simulink model "ThreeSines_DrSaher"  (R2018a)
settings: Solver=FixedStepDiscrete  StartTime=0.0  StopTime=0.1  RelTol=1e-3
InitFcn:
  | ST = 2e-8
  | Ts = 2e-8
libraries: simulink x10, hdlsllib x8, powerlib x1
(part 2 of 2)

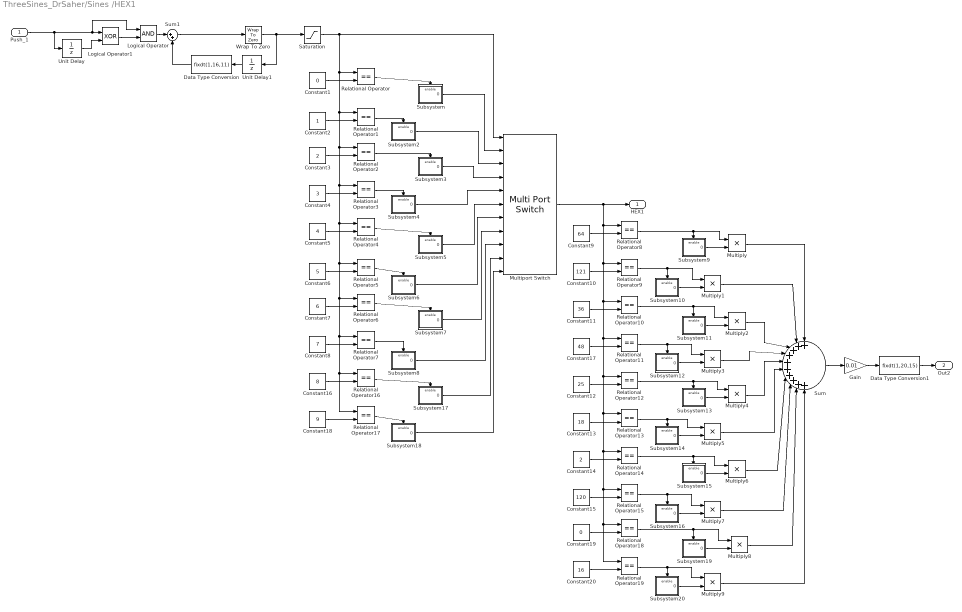
== system ThreeSines_DrSaher/Sines /HEX1 ==
  Push_1 : Inport
  Constant1 : Constant  Value=0  OutMax=[1]  OutDataTypeStr=fixdt(1,16,14)  SampleTime=Ts
  Constant10 : Constant  Value=121  OutMax=[121]  OutDataTypeStr=fixdt(0,7,0)  SampleTime=Ts
  Constant11 : Constant  Value=36  OutMax=[36]  OutDataTypeStr=fixdt(0,7,0)  SampleTime=Ts
  Constant12 : Constant  Value=25  OutMax=[25]  OutDataTypeStr=fixdt(0,7,0)  SampleTime=Ts
  Constant13 : Constant  Value=18  OutMax=[18]  OutDataTypeStr=fixdt(0,7,0)  SampleTime=Ts
  Constant14 : Constant  Value=2  OutMax=[2]  OutDataTypeStr=fixdt(0,7,0)  SampleTime=Ts
  Constant15 : Constant  Value=120  OutMax=[120]  OutDataTypeStr=fixdt(0,7,0)  SampleTime=Ts
  Constant16 : Constant  Value=8  OutMax=[8]  OutDataTypeStr=fixdt(1,16,11)  SampleTime=Ts
  Constant17 : Constant  Value=48  OutMax=[48]  OutDataTypeStr=fixdt(0,7,0)  SampleTime=Ts
  Constant18 : Constant  Value=9  OutMax=[9]  OutDataTypeStr=fixdt(1,16,11)  SampleTime=Ts
  Constant19 : Constant  Value=0  OutMax=[0]  OutDataTypeStr=fixdt(0,7,0)  SampleTime=Ts
  Constant2 : Constant  OutMax=[1]  OutDataTypeStr=fixdt(1,16,14)  SampleTime=Ts
  Constant20 : Constant  Value=16  OutMax=[16]  OutDataTypeStr=fixdt(0,7,0)  SampleTime=Ts
  Constant3 : Constant  Value=2  OutMax=[2]  OutDataTypeStr=fixdt(1,16,13)  SampleTime=Ts
  Constant4 : Constant  Value=3  OutMax=[3]  OutDataTypeStr=fixdt(1,16,13)  SampleTime=Ts
  Constant5 : Constant  Value=4  OutMax=[4]  OutDataTypeStr=fixdt(1,16,12)  SampleTime=Ts
  Constant6 : Constant  Value=5  OutMax=[5]  OutDataTypeStr=fixdt(1,16,12)  SampleTime=Ts
  Constant7 : Constant  Value=6  OutMax=[6]  OutDataTypeStr=fixdt(1,16,12)  SampleTime=Ts
  Constant8 : Constant  Value=7  OutMax=[7]  OutDataTypeStr=fixdt(1,16,12)  SampleTime=Ts
  Constant9 : Constant  Value=64  OutMax=[64]  OutDataTypeStr=fixdt(0,7,0)  SampleTime=Ts
  Data Type Conversion : DataTypeConversion  OutMax=[11]  OutDataTypeStr=fixdt(1,16,11)
  Data Type Conversion1 : DataTypeConversion  OutMin=[0]  OutMax=[0.09]  OutDataTypeStr=fixdt(1,20,15)
  Gain : Gain  Gain=0.01
  Logical Operator : Logic  AllPortsSameDT=off  OutDataTypeStr=boolean
  Logical Operator1 : Logic  Operator=XOR  AllPortsSameDT=off  OutDataTypeStr=boolean
  Multiply{,1..9} (10 alike) : Product
  Multiport Switch : MultiPortSwitch  DataPortOrder=Zero-based contiguous  Inputs=10  zeroidx=on
  Relational Operator{,1..19} (20 alike) : RelationalOperator  Operator===  OutDataTypeStr=boolean  RndMeth=Nearest
  Saturation : Saturate  UpperLimit=9  LowerLimit=0
  Subsystem : Subsystem
  Subsystem10 : Subsystem
  Subsystem11 : Subsystem
  Subsystem12 : Subsystem
  Subsystem13 : Subsystem
  Subsystem14 : Subsystem
  Subsystem15 : Subsystem
  Subsystem16 : Subsystem
  Subsystem17 : Subsystem
  Subsystem18 : Subsystem
  Subsystem19 : Subsystem
  Subsystem2 : Subsystem
  Subsystem20 : Subsystem
  Subsystem3 : Subsystem
  Subsystem4 : Subsystem
  Subsystem5 : Subsystem
  Subsystem6 : Subsystem
  Subsystem7 : Subsystem
  Subsystem8 : Subsystem
  Subsystem9 : Subsystem
  Sum : Sum  Inputs=10
  Sum1 : Sum  Inputs=|++
  Unit Delay : UnitDelay  SampleTime=Ts
  Unit Delay1 : UnitDelay  SampleTime=Ts
  Wrap To Zero : simulink/Discontinuities/Wrap To Zero  Threshold=9
      settings: SourceProductName=Simulink  SourceProductBaseCode=SL
  HEX1 : Outport
  Out2 : Outport  Port=2  OutMax=[0.9]
  wires:
  Sum/1 -> Gain/1
  Data Type Conversion/1 -> Sum1/2
  Wrap To Zero/1 -> Unit Delay1/1, Saturation/1
  Sum1/1 -> Wrap To Zero/1
  Unit Delay1/1 -> Data Type Conversion/1
  Logical Operator/1 -> Sum1/1
  Logical Operator1/1 -> Logical Operator/2
  Unit Delay/1 -> Logical Operator1/2
  Push_1/1 -> Logical Operator1/1, Logical Operator/1, Unit Delay/1
  Saturation/1 -> Multiport Switch/1, Relational Operator17/1, Relational Operator16/1, Relational Operator7/1, Relational Operator6/1, Relational Operator5/1, Relational Operator4/1, Relational Operator3/1, Relational Operator2/1, Relational Operator1/1, Relational Operator/1
  Subsystem17/1(0) -> Multiport Switch/10
  Relational Operator19/1 -> Multiply9/1, Subsystem20/Enable
  Subsystem13/1(0) -> Multiply4/2
  Relational Operator6/1 -> Subsystem7/Enable
  Constant9/1 -> Relational Operator8/2
  Subsystem6/1(0) -> Multiport Switch/7
  Constant14/1 -> Relational Operator14/2
  Relational Operator7/1 -> Subsystem8/Enable
  Relational Operator4/1 -> Subsystem5/Enable
  Relational Operator/1 -> Subsystem/Enable
  Subsystem2/1(0) -> Multiport Switch/3
  Relational Operator15/1 -> Multiply7/1, Subsystem16/Enable
  Multiply4/1 -> Sum/5
  Constant17/1 -> Relational Operator11/2
  Subsystem11/1(0) -> Multiply2/2
  Constant20/1 -> Relational Operator19/2
  Constant8/1 -> Relational Operator7/2
  Multiply9/1 -> Sum/10
  Constant10/1 -> Relational Operator9/2
  Constant13/1 -> Relational Operator13/2
  Subsystem5/1(0) -> Multiport Switch/6
  Subsystem8/1(0) -> Multiport Switch/9
  Relational Operator9/1 -> Subsystem10/Enable, Multiply1/1
  Relational Operator8/1 -> Subsystem9/Enable, Multiply/1
  Constant6/1 -> Relational Operator5/2
  Multiply7/1 -> Sum/8
  Constant15/1 -> Relational Operator15/2
  Multiply6/1 -> Sum/7
  Relational Operator14/1 -> Subsystem15/Enable, Multiply6/1
  Constant18/1 -> Relational Operator17/2
  Relational Operator12/1 -> Subsystem13/Enable, Multiply4/1
  Subsystem14/1(0) -> Multiply5/2
  Subsystem20/1(0) -> Multiply9/2
  Constant7/1 -> Relational Operator6/2
  Constant4/1 -> Relational Operator3/2
  Relational Operator1/1 -> Subsystem2/Enable
  Constant1/1 -> Relational Operator/2
  Relational Operator3/1 -> Subsystem4/Enable
  Relational Operator5/1 -> Subsystem6/Enable
  Subsystem3/1(0) -> Multiport Switch/4
  Constant2/1 -> Relational Operator1/2
  Constant5/1 -> Relational Operator4/2
  Relational Operator2/1 -> Subsystem3/Enable
  Constant12/1 -> Relational Operator12/2
  Multiply2/1 -> Sum/3
  Multiply8/1 -> Sum/9
  Subsystem4/1(0) -> Multiport Switch/5
  Relational Operator17/1 -> Subsystem18/Enable
  Constant3/1 -> Relational Operator2/2
  Subsystem7/1(0) -> Multiport Switch/8
  Constant19/1 -> Relational Operator18/2
  Multiply/1 -> Sum/1
  Multiport Switch/1 -> Relational Operator9/1, Relational Operator10/1, Relational Operator12/1, Relational Operator13/1, Relational Operator14/1, Relational Operator15/1, Relational Operator18/1, Relational Operator19/1, Relational Operator11/1, Relational Operator8/1, HEX1/1
  Multiply5/1 -> Sum/6
  Multiply1/1 -> Sum/2
  Relational Operator11/1 -> Subsystem12/Enable, Multiply3/1
  Constant11/1 -> Relational Operator10/2
  Subsystem12/1(0) -> Multiply3/2
  Subsystem9/1(0) -> Multiply/2
  Subsystem16/1(0) -> Multiply7/2
  Subsystem18/1(0) -> Multiport Switch/11
  Relational Operator13/1 -> Subsystem14/Enable, Multiply5/1
  Subsystem10/1(0) -> Multiply1/2
  Relational Operator18/1 -> Subsystem19/Enable, Multiply8/1
  Multiply3/1 -> Sum/4
  Subsystem19/1(0) -> Multiply8/2
  Subsystem15/1(0) -> Multiply6/2
  Relational Operator16/1 -> Subsystem17/Enable
  Subsystem/1(0) -> Multiport Switch/2
  Constant16/1 -> Relational Operator16/2
  Relational Operator10/1 -> Subsystem11/Enable, Multiply2/1
  Gain/1 -> Data Type Conversion1/1
  Data Type Conversion1/1 -> Out2/1

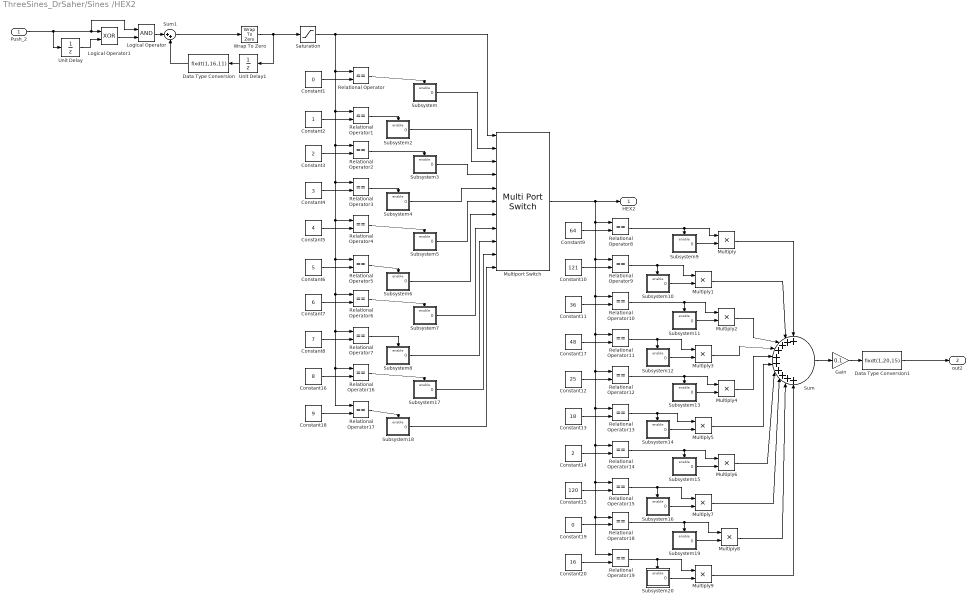
== system ThreeSines_DrSaher/Sines /HEX2 ==
  Push_2 : Inport
  Constant1 : Constant  Value=0  OutMax=[1]  OutDataTypeStr=fixdt(1,16,14)  SampleTime=Ts
  Constant10 : Constant  Value=121  OutMax=[121]  OutDataTypeStr=fixdt(0,7,0)  SampleTime=Ts
  Constant11 : Constant  Value=36  OutMax=[36]  OutDataTypeStr=fixdt(0,7,0)  SampleTime=Ts
  Constant12 : Constant  Value=25  OutMax=[25]  OutDataTypeStr=fixdt(0,7,0)  SampleTime=Ts
  Constant13 : Constant  Value=18  OutMax=[18]  OutDataTypeStr=fixdt(0,7,0)  SampleTime=Ts
  Constant14 : Constant  Value=2  OutMax=[2]  OutDataTypeStr=fixdt(0,7,0)  SampleTime=Ts
  Constant15 : Constant  Value=120  OutMax=[120]  OutDataTypeStr=fixdt(0,7,0)  SampleTime=Ts
  Constant16 : Constant  Value=8  OutMax=[8]  OutDataTypeStr=fixdt(1,16,11)  SampleTime=Ts
  Constant17 : Constant  Value=48  OutMax=[48]  OutDataTypeStr=fixdt(0,7,0)  SampleTime=Ts
  Constant18 : Constant  Value=9  OutMax=[9]  OutDataTypeStr=fixdt(1,16,11)  SampleTime=Ts
  Constant19 : Constant  Value=0  OutMax=[0]  OutDataTypeStr=fixdt(0,7,0)  SampleTime=Ts
  Constant2 : Constant  OutMax=[1]  OutDataTypeStr=fixdt(1,16,14)  SampleTime=Ts
  Constant20 : Constant  Value=16  OutMax=[16]  OutDataTypeStr=fixdt(0,7,0)  SampleTime=Ts
  Constant3 : Constant  Value=2  OutMax=[2]  OutDataTypeStr=fixdt(1,16,13)  SampleTime=Ts
  Constant4 : Constant  Value=3  OutMax=[3]  OutDataTypeStr=fixdt(1,16,13)  SampleTime=Ts
  Constant5 : Constant  Value=4  OutMax=[4]  OutDataTypeStr=fixdt(1,16,12)  SampleTime=Ts
  Constant6 : Constant  Value=5  OutMax=[5]  OutDataTypeStr=fixdt(1,16,12)  SampleTime=Ts
  Constant7 : Constant  Value=6  OutMax=[6]  OutDataTypeStr=fixdt(1,16,12)  SampleTime=Ts
  Constant8 : Constant  Value=7  OutMax=[7]  OutDataTypeStr=fixdt(1,16,12)  SampleTime=Ts
  Constant9 : Constant  Value=64  OutMax=[64]  OutDataTypeStr=fixdt(0,7,0)  SampleTime=Ts
  Data Type Conversion : DataTypeConversion  OutMax=[11]  OutDataTypeStr=fixdt(1,16,11)
  Data Type Conversion1 : DataTypeConversion  OutMin=[0]  OutMax=[0.9]  OutDataTypeStr=fixdt(1,20,15)
  Gain : Gain  Gain=0.1
  Logical Operator : Logic  AllPortsSameDT=off  OutDataTypeStr=boolean
  Logical Operator1 : Logic  Operator=XOR  AllPortsSameDT=off  OutDataTypeStr=boolean
  Multiply{,1..9} (10 alike) : Product
  Multiport Switch : MultiPortSwitch  DataPortOrder=Zero-based contiguous  Inputs=10  zeroidx=on
  Relational Operator{,1..19} (20 alike) : RelationalOperator  Operator===  OutDataTypeStr=boolean  RndMeth=Nearest
  Saturation : Saturate  UpperLimit=9  LowerLimit=0
  Subsystem : Subsystem
  Subsystem10 : Subsystem
  Subsystem11 : Subsystem
  Subsystem12 : Subsystem
  Subsystem13 : Subsystem
  Subsystem14 : Subsystem
  Subsystem15 : Subsystem
  Subsystem16 : Subsystem
  Subsystem17 : Subsystem
  Subsystem18 : Subsystem
  Subsystem19 : Subsystem
  Subsystem2 : Subsystem
  Subsystem20 : Subsystem
  Subsystem3 : Subsystem
  Subsystem4 : Subsystem
  Subsystem5 : Subsystem
  Subsystem6 : Subsystem
  Subsystem7 : Subsystem
  Subsystem8 : Subsystem
  Subsystem9 : Subsystem
  Sum : Sum  Inputs=10
  Sum1 : Sum  Inputs=|++
  Unit Delay : UnitDelay  SampleTime=Ts
  Unit Delay1 : UnitDelay  SampleTime=Ts
  Wrap To Zero : simulink/Discontinuities/Wrap To Zero  Threshold=9
      settings: SourceProductName=Simulink  SourceProductBaseCode=SL
  HEX2 : Outport
  out2 : Outport  Port=2  OutMax=[0.9]
  wires:
  Relational Operator10/1 -> Multiply2/1, Subsystem11/Enable
  Constant16/1 -> Relational Operator16/2
  Subsystem/1(0) -> Multiport Switch/2
  Relational Operator16/1 -> Subsystem17/Enable
  Subsystem15/1(0) -> Multiply6/2
  Subsystem19/1(0) -> Multiply8/2
  Multiply3/1 -> Sum/4
  Relational Operator18/1 -> Multiply8/1, Subsystem19/Enable
  Subsystem10/1(0) -> Multiply1/2
  Relational Operator13/1 -> Multiply5/1, Subsystem14/Enable
  Subsystem18/1(0) -> Multiport Switch/11
  Subsystem16/1(0) -> Multiply7/2
  Subsystem9/1(0) -> Multiply/2
  Subsystem12/1(0) -> Multiply3/2
  Constant11/1 -> Relational Operator10/2
  Relational Operator11/1 -> Multiply3/1, Subsystem12/Enable
  Multiply1/1 -> Sum/2
  Multiply5/1 -> Sum/6
  Multiport Switch/1 -> HEX2/1, Relational Operator8/1, Relational Operator11/1, Relational Operator19/1, Relational Operator18/1, Relational Operator15/1, Relational Operator14/1, Relational Operator13/1, Relational Operator12/1, Relational Operator10/1, Relational Operator9/1
  Multiply/1 -> Sum/1
  Constant19/1 -> Relational Operator18/2
  Subsystem7/1(0) -> Multiport Switch/8
  Constant3/1 -> Relational Operator2/2
  Relational Operator17/1 -> Subsystem18/Enable
  Subsystem4/1(0) -> Multiport Switch/5
  Multiply8/1 -> Sum/9
  Multiply2/1 -> Sum/3
  Constant12/1 -> Relational Operator12/2
  Relational Operator2/1 -> Subsystem3/Enable
  Constant5/1 -> Relational Operator4/2
  Constant2/1 -> Relational Operator1/2
  Subsystem3/1(0) -> Multiport Switch/4
  Relational Operator5/1 -> Subsystem6/Enable
  Relational Operator3/1 -> Subsystem4/Enable
  Constant1/1 -> Relational Operator/2
  Relational Operator1/1 -> Subsystem2/Enable
  Constant4/1 -> Relational Operator3/2
  Constant7/1 -> Relational Operator6/2
  Subsystem20/1(0) -> Multiply9/2
  Subsystem14/1(0) -> Multiply5/2
  Relational Operator12/1 -> Multiply4/1, Subsystem13/Enable
  Constant18/1 -> Relational Operator17/2
  Relational Operator14/1 -> Multiply6/1, Subsystem15/Enable
  Multiply6/1 -> Sum/7
  Constant15/1 -> Relational Operator15/2
  Multiply7/1 -> Sum/8
  Constant6/1 -> Relational Operator5/2
  Relational Operator8/1 -> Multiply/1, Subsystem9/Enable
  Relational Operator9/1 -> Multiply1/1, Subsystem10/Enable
  Subsystem8/1(0) -> Multiport Switch/9
  Subsystem5/1(0) -> Multiport Switch/6
  Constant13/1 -> Relational Operator13/2
  Constant10/1 -> Relational Operator9/2
  Multiply9/1 -> Sum/10
  Constant8/1 -> Relational Operator7/2
  Constant20/1 -> Relational Operator19/2
  Subsystem11/1(0) -> Multiply2/2
  Constant17/1 -> Relational Operator11/2
  Multiply4/1 -> Sum/5
  Relational Operator15/1 -> Subsystem16/Enable, Multiply7/1
  Subsystem2/1(0) -> Multiport Switch/3
  Relational Operator/1 -> Subsystem/Enable
  Relational Operator4/1 -> Subsystem5/Enable
  Relational Operator7/1 -> Subsystem8/Enable
  Constant14/1 -> Relational Operator14/2
  Subsystem6/1(0) -> Multiport Switch/7
  Constant9/1 -> Relational Operator8/2
  Relational Operator6/1 -> Subsystem7/Enable
  Subsystem13/1(0) -> Multiply4/2
  Relational Operator19/1 -> Subsystem20/Enable, Multiply9/1
  Subsystem17/1(0) -> Multiport Switch/10
  Saturation/1 -> Relational Operator/1, Relational Operator1/1, Relational Operator2/1, Relational Operator3/1, Relational Operator4/1, Relational Operator5/1, Relational Operator6/1, Relational Operator7/1, Relational Operator16/1, Relational Operator17/1, Multiport Switch/1
  Push_2/1 -> Unit Delay/1, Logical Operator/1, Logical Operator1/1
  Unit Delay/1 -> Logical Operator1/2
  Logical Operator1/1 -> Logical Operator/2
  Logical Operator/1 -> Sum1/1
  Unit Delay1/1 -> Data Type Conversion/1
  Sum1/1 -> Wrap To Zero/1
  Wrap To Zero/1 -> Saturation/1, Unit Delay1/1
  Data Type Conversion/1 -> Sum1/2
  Sum/1 -> Gain/1
  Gain/1 -> Data Type Conversion1/1
  Data Type Conversion1/1 -> out2/1

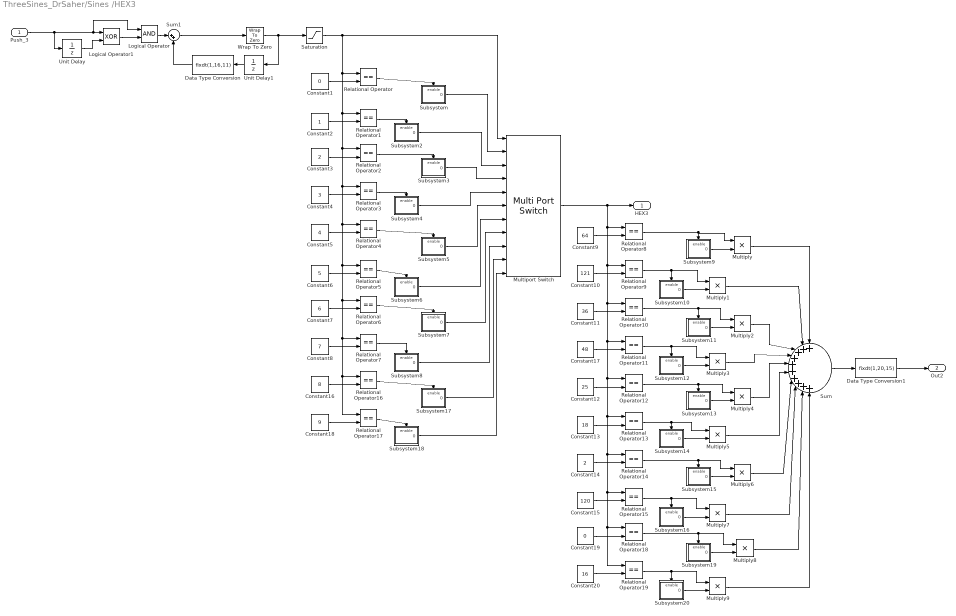
== system ThreeSines_DrSaher/Sines /HEX3 ==
  Push_3 : Inport
  Constant1 : Constant  Value=0  OutMax=[1]  OutDataTypeStr=fixdt(1,16,14)  SampleTime=Ts
  Constant10 : Constant  Value=121  OutMax=[121]  OutDataTypeStr=fixdt(0,7,0)  SampleTime=Ts
  Constant11 : Constant  Value=36  OutMax=[36]  OutDataTypeStr=fixdt(0,7,0)  SampleTime=Ts
  Constant12 : Constant  Value=25  OutMax=[25]  OutDataTypeStr=fixdt(0,7,0)  SampleTime=Ts
  Constant13 : Constant  Value=18  OutMax=[18]  OutDataTypeStr=fixdt(0,7,0)  SampleTime=Ts
  Constant14 : Constant  Value=2  OutMax=[2]  OutDataTypeStr=fixdt(0,7,0)  SampleTime=Ts
  Constant15 : Constant  Value=120  OutMax=[120]  OutDataTypeStr=fixdt(0,7,0)  SampleTime=Ts
  Constant16 : Constant  Value=8  OutMax=[8]  OutDataTypeStr=fixdt(1,16,11)  SampleTime=Ts
  Constant17 : Constant  Value=48  OutMax=[48]  OutDataTypeStr=fixdt(0,7,0)  SampleTime=Ts
  Constant18 : Constant  Value=9  OutMax=[9]  OutDataTypeStr=fixdt(1,16,11)  SampleTime=Ts
  Constant19 : Constant  Value=0  OutMax=[0]  OutDataTypeStr=fixdt(0,7,0)  SampleTime=Ts
  Constant2 : Constant  OutMax=[1]  OutDataTypeStr=fixdt(1,16,14)  SampleTime=Ts
  Constant20 : Constant  Value=16  OutMax=[16]  OutDataTypeStr=fixdt(0,7,0)  SampleTime=Ts
  Constant3 : Constant  Value=2  OutMax=[2]  OutDataTypeStr=fixdt(1,16,13)  SampleTime=Ts
  Constant4 : Constant  Value=3  OutMax=[3]  OutDataTypeStr=fixdt(1,16,13)  SampleTime=Ts
  Constant5 : Constant  Value=4  OutMax=[4]  OutDataTypeStr=fixdt(1,16,12)  SampleTime=Ts
  Constant6 : Constant  Value=5  OutMax=[5]  OutDataTypeStr=fixdt(1,16,12)  SampleTime=Ts
  Constant7 : Constant  Value=6  OutMax=[6]  OutDataTypeStr=fixdt(1,16,12)  SampleTime=Ts
  Constant8 : Constant  Value=7  OutMax=[7]  OutDataTypeStr=fixdt(1,16,12)  SampleTime=Ts
  Constant9 : Constant  Value=64  OutMax=[64]  OutDataTypeStr=fixdt(0,7,0)  SampleTime=Ts
  Data Type Conversion : DataTypeConversion  OutMax=[11]  OutDataTypeStr=fixdt(1,16,11)
  Data Type Conversion1 : DataTypeConversion  OutMin=[0]  OutMax=[9]  OutDataTypeStr=fixdt(1,20,15)
  Logical Operator : Logic  AllPortsSameDT=off  OutDataTypeStr=boolean
  Logical Operator1 : Logic  Operator=XOR  AllPortsSameDT=off  OutDataTypeStr=boolean
  Multiply{,1..9} (10 alike) : Product
  Multiport Switch : MultiPortSwitch  DataPortOrder=Zero-based contiguous  Inputs=10  zeroidx=on
  Relational Operator{,1..19} (20 alike) : RelationalOperator  Operator===  OutDataTypeStr=boolean  RndMeth=Nearest
  Saturation : Saturate  UpperLimit=9  LowerLimit=0
  Subsystem : Subsystem
  Subsystem10 : Subsystem
  Subsystem11 : Subsystem
  Subsystem12 : Subsystem
  Subsystem13 : Subsystem
  Subsystem14 : Subsystem
  Subsystem15 : Subsystem
  Subsystem16 : Subsystem
  Subsystem17 : Subsystem
  Subsystem18 : Subsystem
  Subsystem19 : Subsystem
  Subsystem2 : Subsystem
  Subsystem20 : Subsystem
  Subsystem3 : Subsystem
  Subsystem4 : Subsystem
  Subsystem5 : Subsystem
  Subsystem6 : Subsystem
  Subsystem7 : Subsystem
  Subsystem8 : Subsystem
  Subsystem9 : Subsystem
  Sum : Sum  Inputs=10
  Sum1 : Sum  Inputs=|++
  Unit Delay : UnitDelay  SampleTime=Ts
  Unit Delay1 : UnitDelay  SampleTime=Ts
  Wrap To Zero : simulink/Discontinuities/Wrap To Zero  Threshold=9
      settings: SourceProductName=Simulink  SourceProductBaseCode=SL
  HEX3 : Outport
  Out2 : Outport  Port=2  OutMax=[0.9]
  wires:
  Sum/1 -> Data Type Conversion1/1
  Data Type Conversion/1 -> Sum1/2
  Wrap To Zero/1 -> Unit Delay1/1, Saturation/1
  Sum1/1 -> Wrap To Zero/1
  Unit Delay1/1 -> Data Type Conversion/1
  Logical Operator/1 -> Sum1/1
  Logical Operator1/1 -> Logical Operator/2
  Unit Delay/1 -> Logical Operator1/2
  Push_3/1 -> Logical Operator1/1, Logical Operator/1, Unit Delay/1
  Saturation/1 -> Multiport Switch/1, Relational Operator17/1, Relational Operator16/1, Relational Operator7/1, Relational Operator6/1, Relational Operator5/1, Relational Operator4/1, Relational Operator3/1, Relational Operator2/1, Relational Operator1/1, Relational Operator/1
  Subsystem17/1(0) -> Multiport Switch/10
  Relational Operator19/1 -> Multiply9/1, Subsystem20/Enable
  Subsystem13/1(0) -> Multiply4/2
  Relational Operator6/1 -> Subsystem7/Enable
  Constant9/1 -> Relational Operator8/2
  Subsystem6/1(0) -> Multiport Switch/7
  Constant14/1 -> Relational Operator14/2
  Relational Operator7/1 -> Subsystem8/Enable
  Relational Operator4/1 -> Subsystem5/Enable
  Relational Operator/1 -> Subsystem/Enable
  Subsystem2/1(0) -> Multiport Switch/3
  Relational Operator15/1 -> Multiply7/1, Subsystem16/Enable
  Multiply4/1 -> Sum/5
  Constant17/1 -> Relational Operator11/2
  Subsystem11/1(0) -> Multiply2/2
  Constant20/1 -> Relational Operator19/2
  Constant8/1 -> Relational Operator7/2
  Multiply9/1 -> Sum/10
  Constant10/1 -> Relational Operator9/2
  Constant13/1 -> Relational Operator13/2
  Subsystem5/1(0) -> Multiport Switch/6
  Subsystem8/1(0) -> Multiport Switch/9
  Relational Operator9/1 -> Subsystem10/Enable, Multiply1/1
  Relational Operator8/1 -> Subsystem9/Enable, Multiply/1
  Constant6/1 -> Relational Operator5/2
  Multiply7/1 -> Sum/8
  Constant15/1 -> Relational Operator15/2
  Multiply6/1 -> Sum/7
  Relational Operator14/1 -> Subsystem15/Enable, Multiply6/1
  Constant18/1 -> Relational Operator17/2
  Relational Operator12/1 -> Subsystem13/Enable, Multiply4/1
  Subsystem14/1(0) -> Multiply5/2
  Subsystem20/1(0) -> Multiply9/2
  Constant7/1 -> Relational Operator6/2
  Constant4/1 -> Relational Operator3/2
  Relational Operator1/1 -> Subsystem2/Enable
  Constant1/1 -> Relational Operator/2
  Relational Operator3/1 -> Subsystem4/Enable
  Relational Operator5/1 -> Subsystem6/Enable
  Subsystem3/1(0) -> Multiport Switch/4
  Constant2/1 -> Relational Operator1/2
  Constant5/1 -> Relational Operator4/2
  Relational Operator2/1 -> Subsystem3/Enable
  Constant12/1 -> Relational Operator12/2
  Multiply2/1 -> Sum/3
  Multiply8/1 -> Sum/9
  Subsystem4/1(0) -> Multiport Switch/5
  Relational Operator17/1 -> Subsystem18/Enable
  Constant3/1 -> Relational Operator2/2
  Subsystem7/1(0) -> Multiport Switch/8
  Constant19/1 -> Relational Operator18/2
  Multiply/1 -> Sum/1
  Multiport Switch/1 -> Relational Operator9/1, Relational Operator10/1, Relational Operator12/1, Relational Operator13/1, Relational Operator14/1, Relational Operator15/1, Relational Operator18/1, Relational Operator19/1, Relational Operator11/1, Relational Operator8/1, HEX3/1
  Multiply5/1 -> Sum/6
  Multiply1/1 -> Sum/2
  Relational Operator11/1 -> Subsystem12/Enable, Multiply3/1
  Constant11/1 -> Relational Operator10/2
  Subsystem12/1(0) -> Multiply3/2
  Subsystem9/1(0) -> Multiply/2
  Subsystem16/1(0) -> Multiply7/2
  Subsystem18/1(0) -> Multiport Switch/11
  Relational Operator13/1 -> Subsystem14/Enable, Multiply5/1
  Subsystem10/1(0) -> Multiply1/2
  Relational Operator18/1 -> Subsystem19/Enable, Multiply8/1
  Multiply3/1 -> Sum/4
  Subsystem19/1(0) -> Multiply8/2
  Subsystem15/1(0) -> Multiply6/2
  Relational Operator16/1 -> Subsystem17/Enable
  Subsystem/1(0) -> Multiport Switch/2
  Constant16/1 -> Relational Operator16/2
  Relational Operator10/1 -> Subsystem11/Enable, Multiply2/1
  Data Type Conversion1/1 -> Out2/1

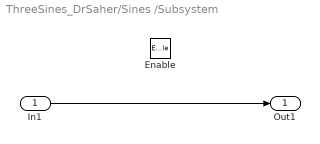
== system ThreeSines_DrSaher/Sines /Subsystem ==
  In1 : Inport
  Enable : EnablePort
  Out1 : Outport  InitialOutput=[0]
  wires:
  In1/1 -> Out1/1

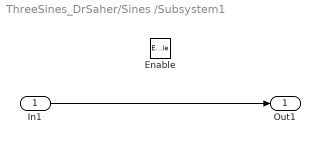
== system ThreeSines_DrSaher/Sines /Subsystem1 ==
  In1 : Inport
  Enable : EnablePort
  Out1 : Outport  InitialOutput=[0]
  wires:
  In1/1 -> Out1/1

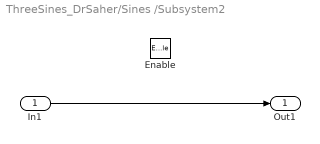
== system ThreeSines_DrSaher/Sines /Subsystem2 ==
  In1 : Inport
  Enable : EnablePort
  Out1 : Outport  InitialOutput=[0]
  wires:
  In1/1 -> Out1/1

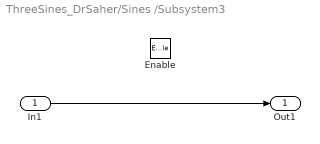
== system ThreeSines_DrSaher/Sines /Subsystem3 ==
  In1 : Inport
  Enable : EnablePort
  Out1 : Outport  InitialOutput=[0]
  wires:
  In1/1 -> Out1/1

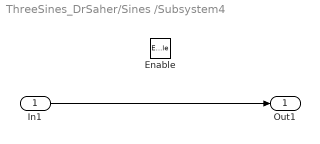
== system ThreeSines_DrSaher/Sines /Subsystem4 ==
  In1 : Inport
  Enable : EnablePort
  Out1 : Outport  InitialOutput=[0]
  wires:
  In1/1 -> Out1/1

== system ThreeSines_DrSaher/Sines /Subsystem5 ==
  In1 : Inport
  Enable : EnablePort
  Out1 : Outport  InitialOutput=[0]
  wires:
  In1/1 -> Out1/1

== system ThreeSines_DrSaher/Sines /Subsystem6 ==
  In1 : Inport
  Enable : EnablePort
  Out1 : Outport  InitialOutput=[0]
  wires:
  In1/1 -> Out1/1

== system ThreeSines_DrSaher/Sines /Subsystem7 ==
  In1 : Inport
  Enable : EnablePort
  Out1 : Outport  InitialOutput=[0]
  wires:
  In1/1 -> Out1/1

== system ThreeSines_DrSaher/Sines /aPA_Save ==
  MulNumber : Inport
  Enable : EnablePort
  MulResult : Outport  InitialOutput=[0]
  wires:
  MulNumber/1 -> MulResult/1

== system ThreeSines_DrSaher/Sines /aPA_Save1 ==
  MulNumber : Inport
  Enable : EnablePort
  MulResult : Outport  InitialOutput=[0]
  wires:
  MulNumber/1 -> MulResult/1

== system ThreeSines_DrSaher/Sines /aPA_Save2 ==
  MulNumber : Inport
  Enable : EnablePort
  MulResult : Outport  InitialOutput=[0]
  wires:
  MulNumber/1 -> MulResult/1

== system ThreeSines_DrSaher/Sines /bPA_Save ==
  MulNumber : Inport
  Enable : EnablePort
  MulResult : Outport  InitialOutput=[0]
  wires:
  MulNumber/1 -> MulResult/1

== system ThreeSines_DrSaher/Sines /bPA_Save1 ==
  MulNumber : Inport
  Enable : EnablePort
  MulResult : Outport  InitialOutput=[0]
  wires:
  MulNumber/1 -> MulResult/1

== system ThreeSines_DrSaher/Sines /bPA_Save2 ==
  MulNumber : Inport
  Enable : EnablePort
  MulResult : Outport  InitialOutput=[0]
  wires:
  MulNumber/1 -> MulResult/1

== system ThreeSines_DrSaher/Sines /cPA_Save ==
  MulNumber : Inport
  Enable : EnablePort
  MulResult : Outport  InitialOutput=[0]
  wires:
  MulNumber/1 -> MulResult/1

== system ThreeSines_DrSaher/Sines /cPA_Save1 ==
  MulNumber : Inport
  Enable : EnablePort
  MulResult : Outport  InitialOutput=[0]
  wires:
  MulNumber/1 -> MulResult/1

== system ThreeSines_DrSaher/Sines /cPA_Save2 ==
  MulNumber : Inport
  Enable : EnablePort
  MulResult : Outport  InitialOutput=[0]
  wires:
  MulNumber/1 -> MulResult/1

== system ThreeSines_DrSaher/Sines /dPA_Save ==
  MulNumber : Inport
  Enable : EnablePort
  MulResult : Outport  InitialOutput=[0]
  wires:
  MulNumber/1 -> MulResult/1

== system ThreeSines_DrSaher/Sines /dPA_Save1 ==
  MulNumber : Inport
  Enable : EnablePort
  MulResult : Outport  InitialOutput=[0]
  wires:
  MulNumber/1 -> MulResult/1

== system ThreeSines_DrSaher/Sines /dPA_Save2 ==
  MulNumber : Inport
  Enable : EnablePort
  MulResult : Outport  InitialOutput=[0]
  wires:
  MulNumber/1 -> MulResult/1

== system ThreeSines_DrSaher/Sines /HEX0/Subsystem ==
  Enable : EnablePort
  Constant9 : Constant  Value=64  OutMax=[64]  OutDataTypeStr=fixdt(0,7,0)  SampleTime=Ts
  0 : Outport  InitialOutput=[0]
  wires:
  Constant9/1 -> 0/1

== system ThreeSines_DrSaher/Sines /HEX0/Subsystem10 ==
  Enable : EnablePort
  Constant9 : Constant  OutMax=[1]  OutDataTypeStr=fixdt(1,16,14)  SampleTime=Ts
  0 : Outport  InitialOutput=[0]
  wires:
  Constant9/1 -> 0/1

== system ThreeSines_DrSaher/Sines /HEX0/Subsystem11 ==
  Enable : EnablePort
  Constant9 : Constant  Value=2  OutMax=[2]  OutDataTypeStr=fixdt(1,16,13)  SampleTime=Ts
  0 : Outport  InitialOutput=[0]
  wires:
  Constant9/1 -> 0/1

== system ThreeSines_DrSaher/Sines /HEX0/Subsystem12 ==
  Enable : EnablePort
  Constant9 : Constant  Value=3  VectorParams1D=off  OutMax=[3]  OutDataTypeStr=fixdt(1,16,13)  SampleTime=Ts
  0 : Outport  InitialOutput=[0]
  wires:
  Constant9/1 -> 0/1

== system ThreeSines_DrSaher/Sines /HEX0/Subsystem13 ==
  Enable : EnablePort
  Constant9 : Constant  Value=4  OutMax=[4]  OutDataTypeStr=fixdt(1,16,12)  SampleTime=Ts
  0 : Outport  InitialOutput=[0]
  wires:
  Constant9/1 -> 0/1

== system ThreeSines_DrSaher/Sines /HEX0/Subsystem14 ==
  Enable : EnablePort
  Constant9 : Constant  Value=5  OutMax=[5]  OutDataTypeStr=fixdt(1,16,12)  SampleTime=Ts
  0 : Outport  InitialOutput=[0]
  wires:
  Constant9/1 -> 0/1

== system ThreeSines_DrSaher/Sines /HEX0/Subsystem15 ==
  Enable : EnablePort
  Constant9 : Constant  Value=6  OutMax=[6]  OutDataTypeStr=fixdt(1,16,12)  SampleTime=Ts
  0 : Outport  InitialOutput=[0]
  wires:
  Constant9/1 -> 0/1

== system ThreeSines_DrSaher/Sines /HEX0/Subsystem16 ==
  Enable : EnablePort
  Constant9 : Constant  Value=7  OutMax=[7]  OutDataTypeStr=fixdt(1,16,12)  SampleTime=Ts
  0 : Outport  InitialOutput=[0]
  wires:
  Constant9/1 -> 0/1

== system ThreeSines_DrSaher/Sines /HEX0/Subsystem17 ==
  Enable : EnablePort
  Constant9 : Constant  Value=0  OutMax=[0]  OutDataTypeStr=fixdt(0,7,0)  SampleTime=Ts
  0 : Outport  InitialOutput=[0]
  wires:
  Constant9/1 -> 0/1

== system ThreeSines_DrSaher/Sines /HEX0/Subsystem18 ==
  Enable : EnablePort
  Constant9 : Constant  Value=16  OutMax=[16]  OutDataTypeStr=fixdt(0,7,0)  SampleTime=Ts
  0 : Outport  InitialOutput=[0]
  wires:
  Constant9/1 -> 0/1

== system ThreeSines_DrSaher/Sines /HEX0/Subsystem19 ==
  Enable : EnablePort
  Constant9 : Constant  Value=8  OutMax=[8]  OutDataTypeStr=fixdt(1,16,11)  SampleTime=Ts
  0 : Outport  InitialOutput=[0]
  wires:
  Constant9/1 -> 0/1

== system ThreeSines_DrSaher/Sines /HEX0/Subsystem2 ==
  Enable : EnablePort
  Constant9 : Constant  Value=121  OutMax=[121]  OutDataTypeStr=fixdt(0,7,0)  SampleTime=Ts
  0 : Outport  InitialOutput=[0]
  wires:
  Constant9/1 -> 0/1

== system ThreeSines_DrSaher/Sines /HEX0/Subsystem20 ==
  Enable : EnablePort
  Constant9 : Constant  Value=9  OutMax=[9]  OutDataTypeStr=fixdt(1,16,11)  SampleTime=Ts
  0 : Outport  InitialOutput=[0]
  wires:
  Constant9/1 -> 0/1

== system ThreeSines_DrSaher/Sines /HEX0/Subsystem3 ==
  Enable : EnablePort
  Constant9 : Constant  Value=36  OutMax=[36]  OutDataTypeStr=fixdt(0,7,0)  SampleTime=Ts
  0 : Outport  InitialOutput=[0]
  wires:
  Constant9/1 -> 0/1

== system ThreeSines_DrSaher/Sines /HEX0/Subsystem4 ==
  Enable : EnablePort
  Constant9 : Constant  Value=48  OutMax=[48]  OutDataTypeStr=fixdt(0,7,0)  SampleTime=Ts
  0 : Outport  InitialOutput=[0]
  wires:
  Constant9/1 -> 0/1

== system ThreeSines_DrSaher/Sines /HEX0/Subsystem5 ==
  Enable : EnablePort
  Constant9 : Constant  Value=25  OutMax=[25]  OutDataTypeStr=fixdt(0,7,0)  SampleTime=Ts
  0 : Outport  InitialOutput=[0]
  wires:
  Constant9/1 -> 0/1

== system ThreeSines_DrSaher/Sines /HEX0/Subsystem6 ==
  Enable : EnablePort
  Constant9 : Constant  Value=18  OutMax=[18]  OutDataTypeStr=fixdt(0,7,0)  SampleTime=Ts
  0 : Outport  InitialOutput=[0]
  wires:
  Constant9/1 -> 0/1

== system ThreeSines_DrSaher/Sines /HEX0/Subsystem7 ==
  Enable : EnablePort
  Constant9 : Constant  Value=2  OutMax=[2]  OutDataTypeStr=fixdt(0,7,0)  SampleTime=Ts
  0 : Outport  InitialOutput=[0]
  wires:
  Constant9/1 -> 0/1

== system ThreeSines_DrSaher/Sines /HEX0/Subsystem8 ==
  Enable : EnablePort
  Constant9 : Constant  Value=120  OutMax=[120]  OutDataTypeStr=fixdt(0,7,0)  SampleTime=Ts
  0 : Outport  InitialOutput=[0]
  wires:
  Constant9/1 -> 0/1

== system ThreeSines_DrSaher/Sines /HEX0/Subsystem9 ==
  Enable : EnablePort
  Constant9 : Constant  Value=0  OutMax=[0]  OutDataTypeStr=fixdt(1,16,10)  SampleTime=Ts
  0 : Outport  InitialOutput=[0]
  wires:
  Constant9/1 -> 0/1

== system ThreeSines_DrSaher/Sines /HEX1/Subsystem ==
  Enable : EnablePort
  Constant9 : Constant  Value=64  OutMax=[64]  OutDataTypeStr=fixdt(0,7,0)  SampleTime=Ts
  0 : Outport  InitialOutput=[0]
  wires:
  Constant9/1 -> 0/1

== system ThreeSines_DrSaher/Sines /HEX1/Subsystem10 ==
  Enable : EnablePort
  Constant9 : Constant  OutMax=[1]  OutDataTypeStr=fixdt(1,16,14)  SampleTime=Ts
  0 : Outport  InitialOutput=[0]
  wires:
  Constant9/1 -> 0/1

== system ThreeSines_DrSaher/Sines /HEX1/Subsystem11 ==
  Enable : EnablePort
  Constant9 : Constant  Value=2  OutMax=[2]  OutDataTypeStr=fixdt(1,16,13)  SampleTime=Ts
  0 : Outport  InitialOutput=[0]
  wires:
  Constant9/1 -> 0/1

== system ThreeSines_DrSaher/Sines /HEX1/Subsystem12 ==
  Enable : EnablePort
  Constant9 : Constant  Value=3  VectorParams1D=off  OutMax=[3]  OutDataTypeStr=fixdt(1,16,13)  SampleTime=Ts
  0 : Outport  InitialOutput=[0]
  wires:
  Constant9/1 -> 0/1

== system ThreeSines_DrSaher/Sines /HEX1/Subsystem13 ==
  Enable : EnablePort
  Constant9 : Constant  Value=4  OutMax=[4]  OutDataTypeStr=fixdt(1,16,12)  SampleTime=Ts
  0 : Outport  InitialOutput=[0]
  wires:
  Constant9/1 -> 0/1

== system ThreeSines_DrSaher/Sines /HEX1/Subsystem14 ==
  Enable : EnablePort
  Constant9 : Constant  Value=5  OutMax=[5]  OutDataTypeStr=fixdt(1,16,12)  SampleTime=Ts
  0 : Outport  InitialOutput=[0]
  wires:
  Constant9/1 -> 0/1

== system ThreeSines_DrSaher/Sines /HEX1/Subsystem15 ==
  Enable : EnablePort
  Constant9 : Constant  Value=6  OutMax=[6]  OutDataTypeStr=fixdt(1,16,12)  SampleTime=Ts
  0 : Outport  InitialOutput=[0]
  wires:
  Constant9/1 -> 0/1

== system ThreeSines_DrSaher/Sines /HEX1/Subsystem16 ==
  Enable : EnablePort
  Constant9 : Constant  Value=7  OutMax=[7]  OutDataTypeStr=fixdt(1,16,12)  SampleTime=Ts
  0 : Outport  InitialOutput=[0]
  wires:
  Constant9/1 -> 0/1

== system ThreeSines_DrSaher/Sines /HEX1/Subsystem17 ==
  Enable : EnablePort
  Constant9 : Constant  Value=0  OutMax=[0]  OutDataTypeStr=fixdt(0,7,0)  SampleTime=Ts
  0 : Outport  InitialOutput=[0]
  wires:
  Constant9/1 -> 0/1

== system ThreeSines_DrSaher/Sines /HEX1/Subsystem18 ==
  Enable : EnablePort
  Constant9 : Constant  Value=16  OutMax=[16]  OutDataTypeStr=fixdt(0,7,0)  SampleTime=Ts
  0 : Outport  InitialOutput=[0]
  wires:
  Constant9/1 -> 0/1

== system ThreeSines_DrSaher/Sines /HEX1/Subsystem19 ==
  Enable : EnablePort
  Constant9 : Constant  Value=8  OutMax=[8]  OutDataTypeStr=fixdt(1,16,11)  SampleTime=Ts
  0 : Outport  InitialOutput=[0]
  wires:
  Constant9/1 -> 0/1

== system ThreeSines_DrSaher/Sines /HEX1/Subsystem2 ==
  Enable : EnablePort
  Constant9 : Constant  Value=121  OutMax=[121]  OutDataTypeStr=fixdt(0,7,0)  SampleTime=Ts
  0 : Outport  InitialOutput=[0]
  wires:
  Constant9/1 -> 0/1

== system ThreeSines_DrSaher/Sines /HEX1/Subsystem20 ==
  Enable : EnablePort
  Constant9 : Constant  Value=9  OutMax=[9]  OutDataTypeStr=fixdt(1,16,11)  SampleTime=Ts
  0 : Outport  InitialOutput=[0]
  wires:
  Constant9/1 -> 0/1

== system ThreeSines_DrSaher/Sines /HEX1/Subsystem3 ==
  Enable : EnablePort
  Constant9 : Constant  Value=36  OutMax=[36]  OutDataTypeStr=fixdt(0,7,0)  SampleTime=Ts
  0 : Outport  InitialOutput=[0]
  wires:
  Constant9/1 -> 0/1

== system ThreeSines_DrSaher/Sines /HEX1/Subsystem4 ==
  Enable : EnablePort
  Constant9 : Constant  Value=48  OutMax=[48]  OutDataTypeStr=fixdt(0,7,0)  SampleTime=Ts
  0 : Outport  InitialOutput=[0]
  wires:
  Constant9/1 -> 0/1

== system ThreeSines_DrSaher/Sines /HEX1/Subsystem5 ==
  Enable : EnablePort
  Constant9 : Constant  Value=25  OutMax=[25]  OutDataTypeStr=fixdt(0,7,0)  SampleTime=Ts
  0 : Outport  InitialOutput=[0]
  wires:
  Constant9/1 -> 0/1

== system ThreeSines_DrSaher/Sines /HEX1/Subsystem6 ==
  Enable : EnablePort
  Constant9 : Constant  Value=18  OutMax=[18]  OutDataTypeStr=fixdt(0,7,0)  SampleTime=Ts
  0 : Outport  InitialOutput=[0]
  wires:
  Constant9/1 -> 0/1

== system ThreeSines_DrSaher/Sines /HEX1/Subsystem7 ==
  Enable : EnablePort
  Constant9 : Constant  Value=2  OutMax=[2]  OutDataTypeStr=fixdt(0,7,0)  SampleTime=Ts
  0 : Outport  InitialOutput=[0]
  wires:
  Constant9/1 -> 0/1

== system ThreeSines_DrSaher/Sines /HEX1/Subsystem8 ==
  Enable : EnablePort
  Constant9 : Constant  Value=120  OutMax=[120]  OutDataTypeStr=fixdt(0,7,0)  SampleTime=Ts
  0 : Outport  InitialOutput=[0]
  wires:
  Constant9/1 -> 0/1

== system ThreeSines_DrSaher/Sines /HEX1/Subsystem9 ==
  Enable : EnablePort
  Constant9 : Constant  Value=0  OutMax=[0]  OutDataTypeStr=fixdt(1,16,10)  SampleTime=Ts
  0 : Outport  InitialOutput=[0]
  wires:
  Constant9/1 -> 0/1

== system ThreeSines_DrSaher/Sines /HEX2/Subsystem ==
  Enable : EnablePort
  Constant9 : Constant  Value=64  OutMax=[64]  OutDataTypeStr=fixdt(0,7,0)  SampleTime=Ts
  0 : Outport  InitialOutput=[0]
  wires:
  Constant9/1 -> 0/1

== system ThreeSines_DrSaher/Sines /HEX2/Subsystem10 ==
  Enable : EnablePort
  Constant9 : Constant  OutMax=[1]  OutDataTypeStr=fixdt(1,16,14)  SampleTime=Ts
  0 : Outport  InitialOutput=[0]
  wires:
  Constant9/1 -> 0/1

== system ThreeSines_DrSaher/Sines /HEX2/Subsystem11 ==
  Enable : EnablePort
  Constant9 : Constant  Value=2  OutMax=[2]  OutDataTypeStr=fixdt(1,16,13)  SampleTime=Ts
  0 : Outport  InitialOutput=[0]
  wires:
  Constant9/1 -> 0/1

== system ThreeSines_DrSaher/Sines /HEX2/Subsystem12 ==
  Enable : EnablePort
  Constant9 : Constant  Value=3  VectorParams1D=off  OutMax=[3]  OutDataTypeStr=fixdt(1,16,13)  SampleTime=Ts
  0 : Outport  InitialOutput=[0]
  wires:
  Constant9/1 -> 0/1

== system ThreeSines_DrSaher/Sines /HEX2/Subsystem13 ==
  Enable : EnablePort
  Constant9 : Constant  Value=4  OutMax=[4]  OutDataTypeStr=fixdt(1,16,12)  SampleTime=Ts
  0 : Outport  InitialOutput=[0]
  wires:
  Constant9/1 -> 0/1

== system ThreeSines_DrSaher/Sines /HEX2/Subsystem14 ==
  Enable : EnablePort
  Constant9 : Constant  Value=5  OutMax=[5]  OutDataTypeStr=fixdt(1,16,12)  SampleTime=Ts
  0 : Outport  InitialOutput=[0]
  wires:
  Constant9/1 -> 0/1

== system ThreeSines_DrSaher/Sines /HEX2/Subsystem15 ==
  Enable : EnablePort
  Constant9 : Constant  Value=6  OutMax=[6]  OutDataTypeStr=fixdt(1,16,12)  SampleTime=Ts
  0 : Outport  InitialOutput=[0]
  wires:
  Constant9/1 -> 0/1

== system ThreeSines_DrSaher/Sines /HEX2/Subsystem16 ==
  Enable : EnablePort
  Constant9 : Constant  Value=7  OutMax=[7]  OutDataTypeStr=fixdt(1,16,12)  SampleTime=Ts
  0 : Outport  InitialOutput=[0]
  wires:
  Constant9/1 -> 0/1

== system ThreeSines_DrSaher/Sines /HEX2/Subsystem17 ==
  Enable : EnablePort
  Constant9 : Constant  Value=0  OutMax=[0]  OutDataTypeStr=fixdt(0,7,0)  SampleTime=Ts
  0 : Outport  InitialOutput=[0]
  wires:
  Constant9/1 -> 0/1

== system ThreeSines_DrSaher/Sines /HEX2/Subsystem18 ==
  Enable : EnablePort
  Constant9 : Constant  Value=16  OutMax=[16]  OutDataTypeStr=fixdt(0,7,0)  SampleTime=Ts
  0 : Outport  InitialOutput=[0]
  wires:
  Constant9/1 -> 0/1

== system ThreeSines_DrSaher/Sines /HEX2/Subsystem19 ==
  Enable : EnablePort
  Constant9 : Constant  Value=8  OutMax=[8]  OutDataTypeStr=fixdt(1,16,11)  SampleTime=Ts
  0 : Outport  InitialOutput=[0]
  wires:
  Constant9/1 -> 0/1

== system ThreeSines_DrSaher/Sines /HEX2/Subsystem2 ==
  Enable : EnablePort
  Constant9 : Constant  Value=121  OutMax=[121]  OutDataTypeStr=fixdt(0,7,0)  SampleTime=Ts
  0 : Outport  InitialOutput=[0]
  wires:
  Constant9/1 -> 0/1

== system ThreeSines_DrSaher/Sines /HEX2/Subsystem20 ==
  Enable : EnablePort
  Constant9 : Constant  Value=9  OutMax=[9]  OutDataTypeStr=fixdt(1,16,11)  SampleTime=Ts
  0 : Outport  InitialOutput=[0]
  wires:
  Constant9/1 -> 0/1

== system ThreeSines_DrSaher/Sines /HEX2/Subsystem3 ==
  Enable : EnablePort
  Constant9 : Constant  Value=36  OutMax=[36]  OutDataTypeStr=fixdt(0,7,0)  SampleTime=Ts
  0 : Outport  InitialOutput=[0]
  wires:
  Constant9/1 -> 0/1

== system ThreeSines_DrSaher/Sines /HEX2/Subsystem4 ==
  Enable : EnablePort
  Constant9 : Constant  Value=48  OutMax=[48]  OutDataTypeStr=fixdt(0,7,0)  SampleTime=Ts
  0 : Outport  InitialOutput=[0]
  wires:
  Constant9/1 -> 0/1

== system ThreeSines_DrSaher/Sines /HEX2/Subsystem5 ==
  Enable : EnablePort
  Constant9 : Constant  Value=25  OutMax=[25]  OutDataTypeStr=fixdt(0,7,0)  SampleTime=Ts
  0 : Outport  InitialOutput=[0]
  wires:
  Constant9/1 -> 0/1

== system ThreeSines_DrSaher/Sines /HEX2/Subsystem6 ==
  Enable : EnablePort
  Constant9 : Constant  Value=18  OutMax=[18]  OutDataTypeStr=fixdt(0,7,0)  SampleTime=Ts
  0 : Outport  InitialOutput=[0]
  wires:
  Constant9/1 -> 0/1

== system ThreeSines_DrSaher/Sines /HEX2/Subsystem7 ==
  Enable : EnablePort
  Constant9 : Constant  Value=2  OutMax=[2]  OutDataTypeStr=fixdt(0,7,0)  SampleTime=Ts
  0 : Outport  InitialOutput=[0]
  wires:
  Constant9/1 -> 0/1

== system ThreeSines_DrSaher/Sines /HEX2/Subsystem8 ==
  Enable : EnablePort
  Constant9 : Constant  Value=120  OutMax=[120]  OutDataTypeStr=fixdt(0,7,0)  SampleTime=Ts
  0 : Outport  InitialOutput=[0]
  wires:
  Constant9/1 -> 0/1

== system ThreeSines_DrSaher/Sines /HEX2/Subsystem9 ==
  Enable : EnablePort
  Constant9 : Constant  Value=0  OutMax=[0]  OutDataTypeStr=fixdt(1,16,10)  SampleTime=Ts
  0 : Outport  InitialOutput=[0]
  wires:
  Constant9/1 -> 0/1

== system ThreeSines_DrSaher/Sines /HEX3/Subsystem ==
  Enable : EnablePort
  Constant9 : Constant  Value=64  OutMax=[64]  OutDataTypeStr=fixdt(0,7,0)  SampleTime=Ts
  0 : Outport  InitialOutput=[0]
  wires:
  Constant9/1 -> 0/1

== system ThreeSines_DrSaher/Sines /HEX3/Subsystem10 ==
  Enable : EnablePort
  Constant9 : Constant  OutMax=[1]  OutDataTypeStr=fixdt(1,16,14)  SampleTime=Ts
  0 : Outport  InitialOutput=[0]
  wires:
  Constant9/1 -> 0/1

== system ThreeSines_DrSaher/Sines /HEX3/Subsystem11 ==
  Enable : EnablePort
  Constant9 : Constant  Value=2  OutMax=[2]  OutDataTypeStr=fixdt(1,16,13)  SampleTime=Ts
  0 : Outport  InitialOutput=[0]
  wires:
  Constant9/1 -> 0/1

== system ThreeSines_DrSaher/Sines /HEX3/Subsystem12 ==
  Enable : EnablePort
  Constant9 : Constant  Value=3  VectorParams1D=off  OutMax=[3]  OutDataTypeStr=fixdt(1,16,13)  SampleTime=Ts
  0 : Outport  InitialOutput=[0]
  wires:
  Constant9/1 -> 0/1

== system ThreeSines_DrSaher/Sines /HEX3/Subsystem13 ==
  Enable : EnablePort
  Constant9 : Constant  Value=4  OutMax=[4]  OutDataTypeStr=fixdt(1,16,12)  SampleTime=Ts
  0 : Outport  InitialOutput=[0]
  wires:
  Constant9/1 -> 0/1

== system ThreeSines_DrSaher/Sines /HEX3/Subsystem14 ==
  Enable : EnablePort
  Constant9 : Constant  Value=5  OutMax=[5]  OutDataTypeStr=fixdt(1,16,12)  SampleTime=Ts
  0 : Outport  InitialOutput=[0]
  wires:
  Constant9/1 -> 0/1

== system ThreeSines_DrSaher/Sines /HEX3/Subsystem15 ==
  Enable : EnablePort
  Constant9 : Constant  Value=6  OutMax=[6]  OutDataTypeStr=fixdt(1,16,12)  SampleTime=Ts
  0 : Outport  InitialOutput=[0]
  wires:
  Constant9/1 -> 0/1

== system ThreeSines_DrSaher/Sines /HEX3/Subsystem16 ==
  Enable : EnablePort
  Constant9 : Constant  Value=7  OutMax=[7]  OutDataTypeStr=fixdt(1,16,12)  SampleTime=Ts
  0 : Outport  InitialOutput=[0]
  wires:
  Constant9/1 -> 0/1

== system ThreeSines_DrSaher/Sines /HEX3/Subsystem17 ==
  Enable : EnablePort
  Constant9 : Constant  Value=0  OutMax=[0]  OutDataTypeStr=fixdt(0,7,0)  SampleTime=Ts
  0 : Outport  InitialOutput=[0]
  wires:
  Constant9/1 -> 0/1

== system ThreeSines_DrSaher/Sines /HEX3/Subsystem18 ==
  Enable : EnablePort
  Constant9 : Constant  Value=16  OutMax=[16]  OutDataTypeStr=fixdt(0,7,0)  SampleTime=Ts
  0 : Outport  InitialOutput=[0]
  wires:
  Constant9/1 -> 0/1

== system ThreeSines_DrSaher/Sines /HEX3/Subsystem19 ==
  Enable : EnablePort
  Constant9 : Constant  Value=8  OutMax=[8]  OutDataTypeStr=fixdt(1,16,11)  SampleTime=Ts
  0 : Outport  InitialOutput=[0]
  wires:
  Constant9/1 -> 0/1

== system ThreeSines_DrSaher/Sines /HEX3/Subsystem2 ==
  Enable : EnablePort
  Constant9 : Constant  Value=121  OutMax=[121]  OutDataTypeStr=fixdt(0,7,0)  SampleTime=Ts
  0 : Outport  InitialOutput=[0]
  wires:
  Constant9/1 -> 0/1

== system ThreeSines_DrSaher/Sines /HEX3/Subsystem20 ==
  Enable : EnablePort
  Constant9 : Constant  Value=9  OutMax=[9]  OutDataTypeStr=fixdt(1,16,11)  SampleTime=Ts
  0 : Outport  InitialOutput=[0]
  wires:
  Constant9/1 -> 0/1

== system ThreeSines_DrSaher/Sines /HEX3/Subsystem3 ==
  Enable : EnablePort
  Constant9 : Constant  Value=36  OutMax=[36]  OutDataTypeStr=fixdt(0,7,0)  SampleTime=Ts
  0 : Outport  InitialOutput=[0]
  wires:
  Constant9/1 -> 0/1

== system ThreeSines_DrSaher/Sines /HEX3/Subsystem4 ==
  Enable : EnablePort
  Constant9 : Constant  Value=48  OutMax=[48]  OutDataTypeStr=fixdt(0,7,0)  SampleTime=Ts
  0 : Outport  InitialOutput=[0]
  wires:
  Constant9/1 -> 0/1

== system ThreeSines_DrSaher/Sines /HEX3/Subsystem5 ==
  Enable : EnablePort
  Constant9 : Constant  Value=25  OutMax=[25]  OutDataTypeStr=fixdt(0,7,0)  SampleTime=Ts
  0 : Outport  InitialOutput=[0]
  wires:
  Constant9/1 -> 0/1

== system ThreeSines_DrSaher/Sines /HEX3/Subsystem6 ==
  Enable : EnablePort
  Constant9 : Constant  Value=18  OutMax=[18]  OutDataTypeStr=fixdt(0,7,0)  SampleTime=Ts
  0 : Outport  InitialOutput=[0]
  wires:
  Constant9/1 -> 0/1

== system ThreeSines_DrSaher/Sines /HEX3/Subsystem7 ==
  Enable : EnablePort
  Constant9 : Constant  Value=2  OutMax=[2]  OutDataTypeStr=fixdt(0,7,0)  SampleTime=Ts
  0 : Outport  InitialOutput=[0]
  wires:
  Constant9/1 -> 0/1

== system ThreeSines_DrSaher/Sines /HEX3/Subsystem8 ==
  Enable : EnablePort
  Constant9 : Constant  Value=120  OutMax=[120]  OutDataTypeStr=fixdt(0,7,0)  SampleTime=Ts
  0 : Outport  InitialOutput=[0]
  wires:
  Constant9/1 -> 0/1

== system ThreeSines_DrSaher/Sines /HEX3/Subsystem9 ==
  Enable : EnablePort
  Constant9 : Constant  Value=0  OutMax=[0]  OutDataTypeStr=fixdt(1,16,10)  SampleTime=Ts
  0 : Outport  InitialOutput=[0]
  wires:
  Constant9/1 -> 0/1
